simulink library "Autonomous_lib"  (R2023a)
settings: Solver=VariableStepAuto  StartTime=0.0  StopTime=10.0  RelTol=1e-3
settings Model: Creator=FIRSTMentor  LastModifiedBy=FIRSTMentor

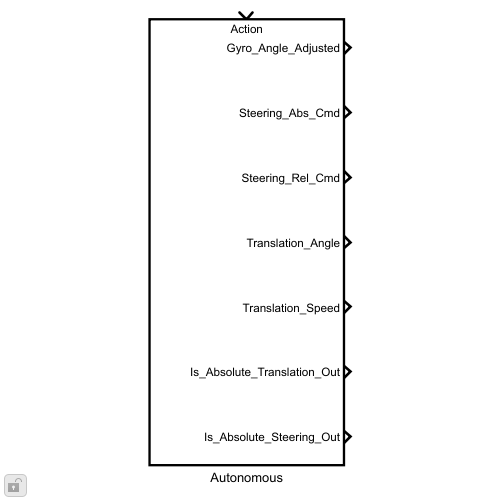
[thumbnail: Simulink's stored preview of the top-level diagram]
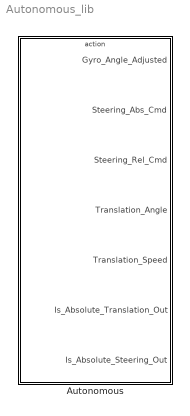
== system Autonomous_lib ==
  Autonomous : Subsystem  TreatAsAtomicUnit=on

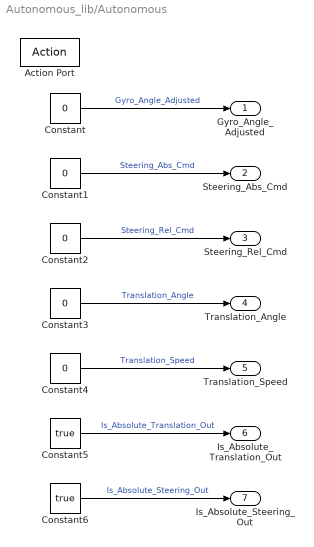
== system Autonomous_lib/Autonomous ==
  Action Port : ActionPort
  Constant{,1..4} (5 alike) : Constant  Value=0
  Constant5 : Constant  Value=true
  Constant6 : Constant  Value=true
  Gyro_Angle_Adjusted : Outport
  Steering_Abs_Cmd : Outport  Port=2
  Steering_Rel_Cmd : Outport  Port=3
  Translation_Angle : Outport  Port=4
  Translation_Speed : Outport  Port=5
  Is_Absolute_Translation_Out : Outport  Port=6
  Is_Absolute_Steering_Out : Outport  Port=7
  wires:
  Constant1/1 -> Steering_Abs_Cmd/1  "Steering_Abs_Cmd"
  Constant2/1 -> Steering_Rel_Cmd/1  "Steering_Rel_Cmd"
  Constant3/1 -> Translation_Angle/1  "Translation_Angle"
  Constant/1 -> Gyro_Angle_Adjusted/1  "Gyro_Angle_Adjusted"
  Constant5/1 -> Is_Absolute_Translation_Out/1  "Is_Absolute_Translation_Out"
  Constant4/1 -> Translation_Speed/1  "Translation_Speed"
  Constant6/1 -> Is_Absolute_Steering_Out/1  "Is_Absolute_Steering_Out"
